simulink model "FLC_control"  (R2020a)
settings: Solver=VariableStepAuto  StartTime=0.0  StopTime=10.0  RelTol=1e-3
values from neighbouring files (symbols this model uses):
  B = .1    (= 0.1)    [parameters.m]
  J = .01    (= 0.01)    [parameters.m]
  K = .01    (= 0.01)    [parameters.m]
  L = .5    (= 0.5)    [parameters.m]
  R = 1    [parameters.m]
libraries: fuzblock x1
settings Model: Creator=Maria  LastModifiedBy=Maria

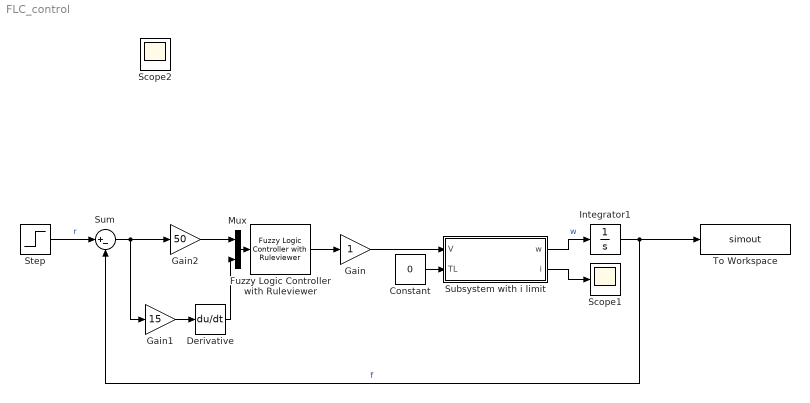
== system FLC_control ==
  Constant : Constant  Value=0
  Derivative : Derivative
  Fuzzy Logic Controller with Ruleviewer : fuzblock/Fuzzy Logic  Controller  with Ruleviewer  fismatrix=FLC_control  Ts=0.25
  Gain : Gain
  Gain1 : Gain  Gain=15
  Gain2 : Gain  Gain=50
  Integrator1 : Integrator
  Mux : Mux  Inputs=2
  Scope1 : Scope
  Step : Step  Time=0  SampleTime=0
  Subsystem with i limit : Subsystem
  Sum : Sum  Inputs=|+-
  To Workspace : ToWorkspace  VariableName=simout  SaveFormat=Timeseries  SampleTime=-1
  Scope2 : Scope
  wires:
  Integrator1/1 -> To Workspace/1, Sum/2  "f"
  Step/1 -> Sum/1  "r"
  Subsystem with i limit/1(w) -> Integrator1/1  "w"
  Gain/1 -> Subsystem with i limit/1(V)
  Constant/1 -> Subsystem with i limit/2(TL)
  Subsystem with i limit/2(i) -> Scope1/1
  Fuzzy Logic Controller with Ruleviewer/1 -> Gain/1
  Mux/1 -> Fuzzy Logic Controller with Ruleviewer/1
  Sum/1 -> Gain1/1, Gain2/1
  Gain2/1 -> Mux/1
  Gain1/1 -> Derivative/1
  Derivative/1 -> Mux/2

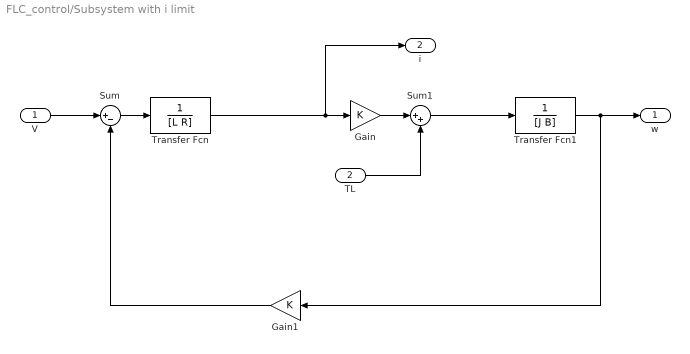
== system FLC_control/Subsystem with i limit ==
  V : Inport
  TL : Inport  Port=2
  Gain : Gain  Gain=K
  Gain1 : Gain  Gain=K
  Sum : Sum  Inputs=|+-
  Sum1 : Sum  Inputs=|++
  Transfer Fcn : TransferFcn  Denominator=[L R]
  Transfer Fcn1 : TransferFcn  Denominator=[J B]
  w : Outport  VectorParamsAs1DForOutWhenUnconnected=off
  i : Outport  Port=2  VectorParamsAs1DForOutWhenUnconnected=off
  wires:
  Transfer Fcn1/1 -> w/1, Gain1/1
  Gain1/1 -> Sum/2
  V/1 -> Sum/1
  Sum/1 -> Transfer Fcn/1
  Gain/1 -> Sum1/1
  Sum1/1 -> Transfer Fcn1/1
  TL/1 -> Sum1/2
  Transfer Fcn/1 -> Gain/1, i/1
